simulink model "SM_Euge"  (R2021a)
settings: Solver=VariableStepAuto  StartTime=0.0  StopTime=10000  FixedStep=0.001  RelTol=1e-3
undefined symbols (not defined in the file): Earth, WGS84
libraries: sharedtransform x2, aerolib6dof2 x1
settings Model: Creator=Euge Etcheverry  LastModifiedBy=Euge Etcheverry

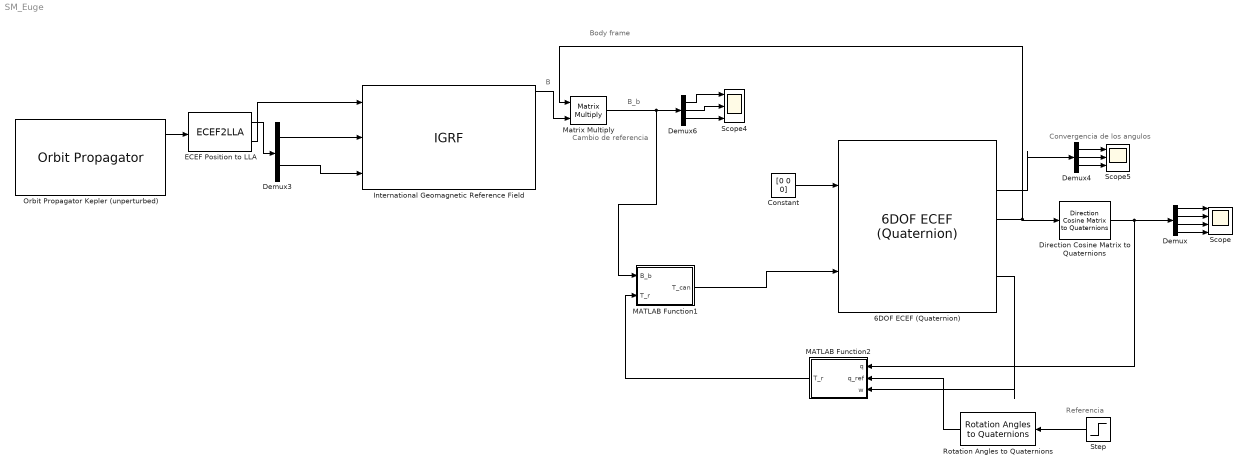
== system SM_Euge ==
  note: Body frame
  note: B
  note: B_b
  note: Cambio de referencia
  note: Referencia
  note: Convergencia de los angulos
  6DOF ECEF (Quaternion) : aerolib6dof2/6DOF ECEF (Quaternion)  units=Metric (MKS)  mtype=Fixed  xg_0=[0 0 0]  Vm_0=[0 0 0]  eul_0="[0  0 0]"  pm_0=[0 0 0]  mass_0=1.0  mass_e=0.5  mass_f=2.0  inertia=2e-3*eye(3)  inertia_e=eye(3)  inertia_f=2*eye(3)  vre_flag=on  abi_flag=off  ptype=Earth (WGS84)  R=6378137  F=1/298.257223563  w_E=7292115e-11  angle_in=Internal  LG0=0  quat_statename=''  pm_statename=''  Vm_statename=''  posECEF_statename=''  posECI_statename=''  LG_statename=''  mass_statename=''
      settings: SourceProductBaseCode=AE
  Constant : Constant  Value=[0 0 0]
  Demux : Demux
  Demux3 : Demux  Outputs=2
  Demux4 : Demux  Outputs=3
  Demux6 : Demux  Outputs=3
  Direction Cosine Matrix to Quaternions : sharedtransform/Direction Cosine Matrix  to Quaternions  aMode=0  action=None  tolerance=eps(2)
      settings: SourceProductBaseCode=AE,PW,DR,MT,UV,VE
  ECEF Position to LLA : ECEF2LLA
  International Geomagnetic Reference Field : IGRF  time_in=off  month=February  day=23  year=2024
      settings: AttributesFormatString=%<generation>
  MATLAB Function1 : MATLAB Function  TreatAsAtomicUnit=on
  MATLAB Function2 : MATLAB Function  TreatAsAtomicUnit=on
  Matrix Multiply : Product  Multiplication=Matrix(*)
  Orbit Propagator Kepler (unperturbed) : OrbitPropagator  startDate=[2024, 02, 23, 12, 32, 16]  eccentricity=0.0005  inclination=98.06  raan=105  trueAnomaly=180  customMu=4.305e13  customJ2=1.0826269e-03  timeFormat=Gregorian
  Rotation Angles to Quaternions : sharedtransform/Rotation Angles to Quaternions  rotationOrder=ZYX  aMode=aMode
      settings: SourceProductBaseCode=AE,PW,DR,MT,UV,VE
  Scope : Scope  NumInputPorts=4
  Scope4 : Scope  NumInputPorts=3
  Scope5 : Scope  NumInputPorts=3
  Step : Step  Before=[0, 0, 0]  After=[0, 0.8, 0.8]  SampleTime=0
  wires:
  6DOF ECEF (Quaternion)/6 -> Matrix Multiply/1, Direction Cosine Matrix to Quaternions/1
  Direction Cosine Matrix to Quaternions/1 -> MATLAB Function2/1(q), Demux/1
  Demux/1 -> Scope/1
  Demux/3 -> Scope/3
  Demux/4 -> Scope/4
  Demux/2 -> Scope/2
  Rotation Angles to Quaternions/1 -> MATLAB Function2/2(q_ref)
  Demux4/1 -> Scope5/1
  Demux4/2 -> Scope5/2
  Demux4/3 -> Scope5/3
  6DOF ECEF (Quaternion)/4 -> Demux4/1
  ECEF Position to LLA/1 -> Demux3/1
  Orbit Propagator Kepler (unperturbed)/1 -> ECEF Position to LLA/1
  Step/1 -> Rotation Angles to Quaternions/1
  International Geomagnetic Reference Field/1 -> Matrix Multiply/2
  Matrix Multiply/1 -> MATLAB Function1/1(B_b), Demux6/1
  Constant/1 -> 6DOF ECEF (Quaternion)/1
  Demux6/1 -> Scope4/1
  Demux6/2 -> Scope4/2
  Demux6/3 -> Scope4/3
  ECEF Position to LLA/2 -> International Geomagnetic Reference Field/1
  Demux3/1 -> International Geomagnetic Reference Field/2
  Demux3/2 -> International Geomagnetic Reference Field/3
  MATLAB Function2/1(T_r) -> MATLAB Function1/2(T_r)
  MATLAB Function1/1(T_can) -> 6DOF ECEF (Quaternion)/2
  6DOF ECEF (Quaternion)/10 -> MATLAB Function2/3(w)

== matlab function SM_Euge/MATLAB Function2 ==
  data: q input; q_ref input; T_r output; w input
function T_r = fcn(q,q_ref, w)
%Inertia
I_xx = 2e-3;
I_yy = 2e-3;
I_zz = 2e-3;
%Error between the quaternions
%Calculate relative quaternion (q2 * inv(q1))
q_error = zeros(1,4); 
q_error = quatmultiply(q_ref, quatinv(q));
%Persistent variable to store previous error
persistent e_prev
if isempty(e_prev)
   e_prev = [0 0 0 0];
end 
dt = 10e-3; %Sampling time
a = 1;
%Sliding surface
q_diff = quatmultiply(q_error, quatinv(e_prev))
sj = q_diff(3)/dt + a*q_error(3);
sk = q_diff(4)/dt + a*q_error(4);
%Save in memory
e_prev = q_error;
%Dynamics 
f_j = -((I_xx - I_zz)/I_yy)*w(3)*w(1);
f_k = -((I_yy - I_xx)/I_zz)*w(2)*w(1);
%Input 
g_j = 1/I_yy;
g_k = 1/I_zz;
% Control law: u = -inv(Cg) * Cf
% Sliding matrix C = [0 0 1 0 0 a 0; 0 0 0 1 0 0 a]
% Only affects uj and uk, so reduced to:
Cg = [g_j 0; 0 g_k];
Cf = [f_j + a * 0; f_k + a * 0];  % No time deriv of w_j, w_k here
% Control torques (only j and k)
u_jk = -Cg \ Cf;
% Assemble total torque vector
T_r = [0 u_jk(1) u_jk(2)];

== matlab function SM_Euge/MATLAB Function1 ==
  data: B_b input; T_can output; T_r input
function T_can = fcn(B_b, T_r)
    B_escalado = B_b * 1e-9;
    %B_norm = norm(B_escalado);
    %if B_norm < 1e-12 %Por si es muy chico
        %T_can = [0; 0; 0];
        %return;
    %end
   % M = cross(B_escalado, T_r)/(B_norm^2);
    %Limites de saturacion del momento magnetico
   % M(3) = 0;
    %M_max = 0.2;
    %for i = 2:3
        %if M(i) > M_max
        %    M(i) = M_max;
        %elseif M(i) < -M_max
         %   M(i) = -M_max;
        %end
    %end
    %T_can = cross(M, B_escalado);
    %T_can(3) = 0;
    %Se que T = M x B y que como queremos controlar Z, Mz = 0
    M = [0; 0; 0];
    M(1) = -T_r(2)/(B_escalado(3));
    M(2) = T_r(1)/(B_escalado(3));
    M(3) = 0;
    M_max = 0.2;
    for i = 1:2
        if M(i) > M_max
            M(i) = M_max;
        elseif M(i) < -M_max
            M(i) = -M_max;
        end
    end
    T_can = cross(M, B_escalado);
    T_can(3) = 0;
end
